simulink library "PM100DX"  (R2024a)
settings: Solver=VariableStepAuto  StartTime=0.0  StopTime=10.0  RelTol=1e-3
undefined symbols (not defined in the file): raptor_xcp_function, StateCAN
libraries: Utilities x10, Raptor_lib x4, simulink x1
settings Model: Creator=serga  LastModifiedBy=serga

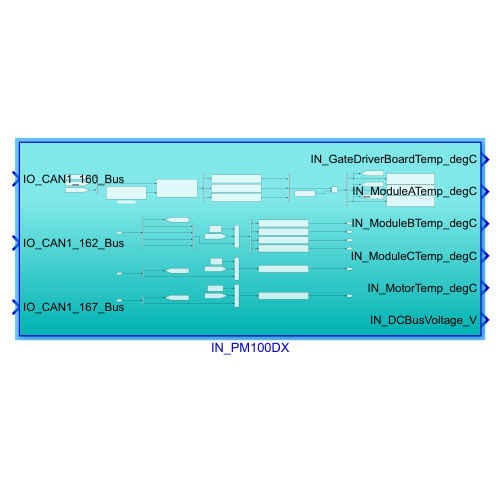
[thumbnail: Simulink's stored preview of the top-level diagram]
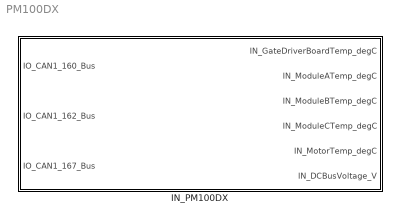
== system PM100DX ==
  IN_PM100DX : Subsystem

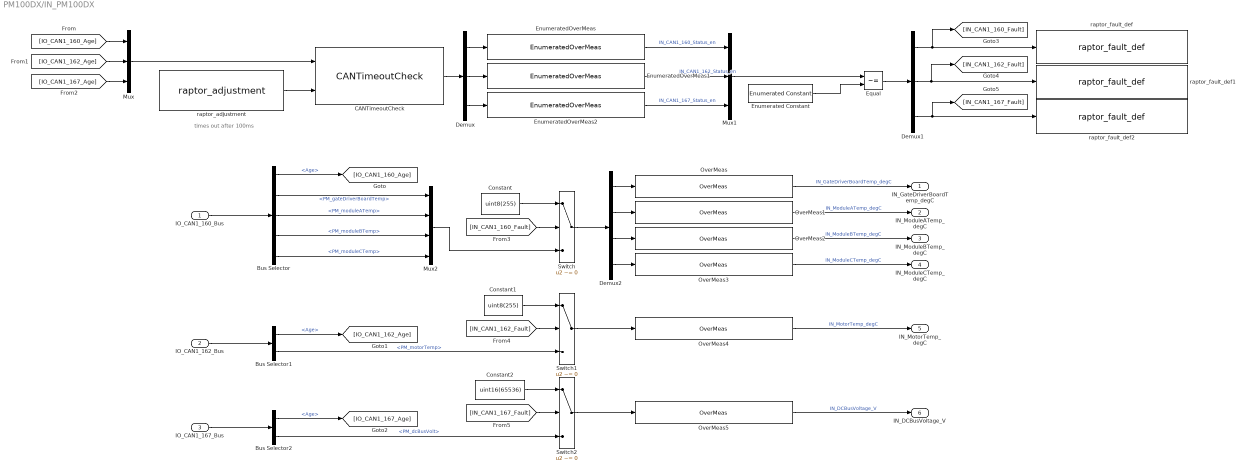
== system PM100DX/IN_PM100DX ==
  note: times out after 100ms
  IO_CAN1_160_Bus : Inport
  IO_CAN1_162_Bus : Inport  Port=2
  IO_CAN1_167_Bus : Inport  Port=3
  Bus Selector : BusSelector  OutputSignals=Age,PM_gateDriverBoardTemp,PM_moduleATemp,PM_moduleBTemp,PM_moduleCTemp
  Bus Selector1 : BusSelector  OutputSignals=Age,PM_motorTemp
  Bus Selector2 : BusSelector  OutputSignals=Age,PM_dcBusVolt
  CANTimeoutCheck : Utilities/CANTimeoutCheck
  Constant : Constant  Value=uint8(255)
  Constant1 : Constant  Value=uint8(255)
  Constant2 : Constant  Value=uint16(65536)
  Demux : Demux  Outputs=3
  Demux1 : Demux  Outputs=3
  Demux2 : Demux
  Enumerated Constant : simulink/Sources/Enumerated Constant  OutDataTypeStr=Enum: StateCAN  Value=StateCAN.Normal  SampleTime=inf
  EnumeratedOverMeas : Utilities/EnumeratedOverMeas  sigName='IN_CAN1_160_Status_en'  enumName='StateCAN'
  EnumeratedOverMeas1 : Utilities/EnumeratedOverMeas  sigName='IN_CAN1_162_Status_en'  enumName='StateCAN'
  EnumeratedOverMeas2 : Utilities/EnumeratedOverMeas  sigName='IN_CAN1_167_Status_en'  enumName='StateCAN'
  Equal : RelationalOperator  Operator=~=  OutDataTypeStr=boolean  RndMeth=Simplest  InputSameDT=off
  Mux : Mux  Inputs=3
  Mux1 : Mux  Inputs=3
  Mux2 : Mux
  OverMeas : Utilities/OverMeas  sigName='IN_GateDriverBoardTemp_degC'  minimum=-inf  maximum=inf
  OverMeas1 : Utilities/OverMeas  sigName='IN_ModuleATemp_degC'  minimum=-inf  maximum=inf
  OverMeas2 : Utilities/OverMeas  sigName='IN_ModuleBTemp_degC'  minimum=-inf  maximum=inf
  OverMeas3 : Utilities/OverMeas  sigName='IN_ModuleCTemp_degC'  minimum=-inf  maximum=inf
  OverMeas4 : Utilities/OverMeas  sigName='IN_MotorTemp_degC'  minimum=-128  maximum=127
  OverMeas5 : Utilities/OverMeas  sigName='IN_DCBusVoltage_V'  minimum=-inf  maximum=inf
  Switch : Switch  Criteria=u2 ~= 0  SaturateOnIntegerOverflow=off  InputSameDT=off
  Switch1 : Switch  Criteria=u2 ~= 0  SaturateOnIntegerOverflow=off  InputSameDT=off
  Switch2 : Switch  Criteria=u2 ~= 0  SaturateOnIntegerOverflow=off  InputSameDT=off
  raptor_adjustment : Raptor_lib/Data Storage/raptor_adjustment  paramName='IN_PM100DXTOThresh_na'  nameSource=Parameter  initValue=20  dataType=uint32  storage=Calibration  calDispType=Number  calEnum={'False', 'True'}  calGain=1.0  calOffset=0.0  calMax=inf  calMin=-inf  calFormat='-1'  calUnit=''  calHelp=''  calAccess=1  calFunction=raptor_xcp_function(gcb)  calDispHeaders=off  calColHeaders={'Col1' 'Col2' 'Col3'}  calRowHeaders={'Row1' 'Row2' 'Row3'}
      settings: SourceProductName=Raptor
  raptor_fault_def : Raptor_lib/Faults/raptor_fault_def  faultName='IN_CAN1_160_Fault'  persist=on  sticky=off  emisRelated=off  singleTrip=off  clearMethod=Standard  xLimit=25  yLimit=50  calEnable=on  addDisable=off  calAccess=1  calFunction='System | FaultManager'
      settings: SourceProductName=Raptor
  raptor_fault_def1 : Raptor_lib/Faults/raptor_fault_def  faultName='IN_CAN1_162_Fault'  persist=on  sticky=off  emisRelated=off  singleTrip=off  clearMethod=Standard  xLimit=25  yLimit=50  calEnable=on  addDisable=off  calAccess=1  calFunction='System | FaultManager'
      settings: SourceProductName=Raptor
  raptor_fault_def2 : Raptor_lib/Faults/raptor_fault_def  faultName='IN_CAN1_167_Fault'  persist=on  sticky=off  emisRelated=off  singleTrip=off  clearMethod=Standard  xLimit=25  yLimit=50  calEnable=on  addDisable=off  calAccess=1  calFunction='System | FaultManager'
      settings: SourceProductName=Raptor
  IN_GateDriverBoardTemp_degC : Outport
  IN_ModuleATemp_degC : Outport  Port=2
  IN_ModuleBTemp_degC : Outport  Port=3
  IN_ModuleCTemp_degC : Outport  Port=4
  IN_MotorTemp_degC : Outport  Port=5
  IN_DCBusVoltage_V : Outport  Port=6
  wires:
  OverMeas5/1 -> IN_DCBusVoltage_V/1  "IN_DCBusVoltage_V"
  Constant2/1 -> Switch2/1
  [IN_CAN1_167_Fault] -> Switch2/2
  OverMeas4/1 -> IN_MotorTemp_degC/1  "IN_MotorTemp_degC"
  Switch1/1 -> OverMeas4/1
  Constant1/1 -> Switch1/1
  [IN_CAN1_162_Fault] -> Switch1/2
  OverMeas3/1 -> IN_ModuleCTemp_degC/1  "IN_ModuleCTemp_degC"
  OverMeas2/1 -> IN_ModuleBTemp_degC/1  "IN_ModuleBTemp_degC"
  OverMeas1/1 -> IN_ModuleATemp_degC/1  "IN_ModuleATemp_degC"
  OverMeas/1 -> IN_GateDriverBoardTemp_degC/1  "IN_GateDriverBoardTemp_degC"
  Demux2/4 -> OverMeas3/1
  Demux2/3 -> OverMeas2/1
  Demux2/2 -> OverMeas1/1
  Demux2/1 -> OverMeas/1
  Switch/1 -> Demux2/1
  Constant/1 -> Switch/1
  [IN_CAN1_160_Fault] -> Switch/2
  Mux2/1 -> Switch/3
  Demux1/3 -> [IN_CAN1_167_Fault], raptor_fault_def2/1
  Demux1/2 -> [IN_CAN1_162_Fault], raptor_fault_def1/1
  Demux1/1 -> [IN_CAN1_160_Fault], raptor_fault_def/1
  Equal/1 -> Demux1/1
  Mux1/1 -> Equal/1
  EnumeratedOverMeas2/1 -> Mux1/3  "IN_CAN1_167_Status_en"
  EnumeratedOverMeas1/1 -> Mux1/2  "IN_CAN1_162_Status_en"
  EnumeratedOverMeas/1 -> Mux1/1  "IN_CAN1_160_Status_en"
  Demux/3 -> EnumeratedOverMeas2/1
  Demux/2 -> EnumeratedOverMeas1/1
  Demux/1 -> EnumeratedOverMeas/1
  Enumerated Constant/1 -> Equal/2
  CANTimeoutCheck/1 -> Demux/1
  raptor_adjustment/1 -> CANTimeoutCheck/2
  [IO_CAN1_167_Age] -> Mux/3
  [IO_CAN1_162_Age] -> Mux/2
  [IO_CAN1_160_Age] -> Mux/1
  Mux/1 -> CANTimeoutCheck/1
  Bus Selector2/2 -> Switch2/3  "<PM_dcBusVolt>"
  Bus Selector2/1 -> [IO_CAN1_167_Age]  "<Age>"
  Bus Selector1/2 -> Switch1/3  "<PM_motorTemp>"
  Bus Selector1/1 -> [IO_CAN1_162_Age]  "<Age>"
  Bus Selector/5 -> Mux2/4  "<PM_moduleCTemp>"
  Bus Selector/4 -> Mux2/3  "<PM_moduleBTemp>"
  Bus Selector/3 -> Mux2/2  "<PM_moduleATemp>"
  Bus Selector/2 -> Mux2/1  "<PM_gateDriverBoardTemp>"
  Bus Selector/1 -> [IO_CAN1_160_Age]  "<Age>"
  IO_CAN1_160_Bus/1 -> Bus Selector/1
  IO_CAN1_162_Bus/1 -> Bus Selector1/1
  IO_CAN1_167_Bus/1 -> Bus Selector2/1
  Switch2/1 -> OverMeas5/1
